simulink model "secondcw"  (R2017a)
settings: Solver=VariableStepAuto  StartTime=0.0  StopTime=10  RelTol=1e-3
settings Model: Creator=RIC  LastModifiedBy=RIC

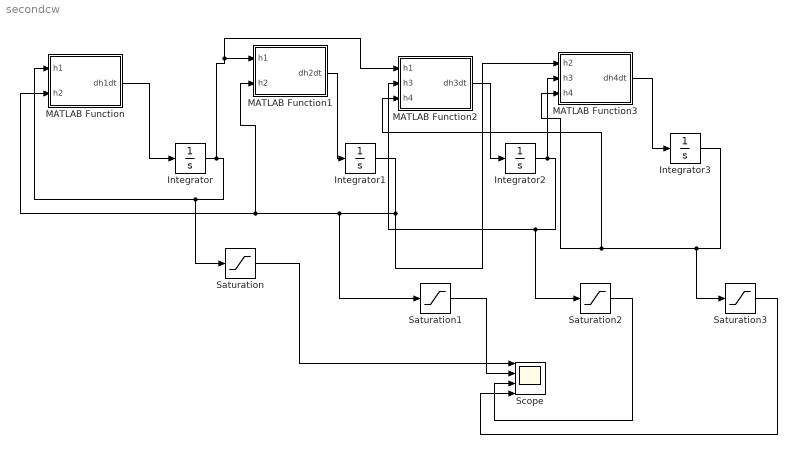
== system secondcw ==
  Integrator{,1..3} (4 alike) : Integrator
  MATLAB Function : MATLAB Function  TreatAsAtomicUnit=on
  MATLAB Function1 : MATLAB Function  TreatAsAtomicUnit=on
  MATLAB Function2 : MATLAB Function  TreatAsAtomicUnit=on
  MATLAB Function3 : MATLAB Function  TreatAsAtomicUnit=on
  Saturation{,1..3} (4 alike) : Saturate  UpperLimit=6  LowerLimit=0
  Scope : Scope  NumInputPorts=4
  wires:
  MATLAB Function/1(dh1dt) -> Integrator/1
  Integrator/1 -> MATLAB Function2/1(h1), MATLAB Function1/1(h1), Saturation/1, MATLAB Function/1(h1)
  MATLAB Function1/1(dh2dt) -> Integrator1/1
  Integrator1/1 -> MATLAB Function3/1(h2), Saturation1/1, MATLAB Function/2(h2), MATLAB Function1/2(h2)
  MATLAB Function2/1(dh3dt) -> Integrator2/1
  Integrator2/1 -> MATLAB Function3/2(h3), Saturation2/1, MATLAB Function2/2(h3)
  MATLAB Function3/1(dh4dt) -> Integrator3/1
  Integrator3/1 -> Saturation3/1, MATLAB Function2/3(h4), MATLAB Function3/3(h4)
  Saturation/1 -> Scope/1
  Saturation1/1 -> Scope/2
  Saturation2/1 -> Scope/3
  Saturation3/1 -> Scope/4

== matlab function secondcw/MATLAB Function1 ==
  data: h1 input; dh2dt output; h2 input
function dh2dt = fcn(h1,h2)
A=pi*.566^2/4;
q2=10;
q1h= 2.5*(h1-h2);
q2v=5*h2;

dh2dt=(q2+q1h-q2v)/A;

== matlab function secondcw/MATLAB Function ==
  data: h1 input; dh1dt output; h2 input
function dh1dt = fcn(h1,h2)
A=pi*.566^2/4;
q1=15;
q1h= 2.5*(h1-h2);
q1v=5*h1;

dh1dt=(q1-q1h-q1v)/A;

== matlab function secondcw/MATLAB Function2 ==
  data: h1 input; dh3dt output; h3 input; h4 input
function dh3dt = fcn(h1,h3,h4)
A=pi*.566^2/4;

q3h= 2.5*(h3-h4);
q1v=5*h1;

dh3dt=(q1v-q3h)/A;

== matlab function secondcw/MATLAB Function3 ==
  data: h2 input; h3 input; dh4dt output; h4 input
function dh4dt = fcn(h2,h3,h4)
A=pi*.566^2/4;

q2v=5*h2;
q4h=2.5*h4;
q3h= 2.5*(h3-h4);
dh4dt=(q2v+q3h-q4h)/A;
